simulink model "car_dynamics"  (R2023a)
settings: Solver=ode1be  StartTime=0.0  StopTime=100  FixedStep=0.01  RelTol=1e-4  AbsTol=1e-4
libraries: simulink_extras x3
settings Model: Creator=Sebas  LastModifiedBy=maxpr
settings SolverCC: AutoScaleAbsTol=off  SolverJacobianMethodControl=SparsePerturbation  AlgebraicLoopSolver=TrustRegion  EnableFixedStepZeroCrossing=on
settings OptimizationCC: ReuseModelBlockBuffer=off
settings DebuggingCC: UnconnectedInputMsg=warning  UnconnectedOutputMsg=warning  UnconnectedLineMsg=warning
settings ModelReferenceCC: EnableRefExpFcnMdlSchedulingChecks=on

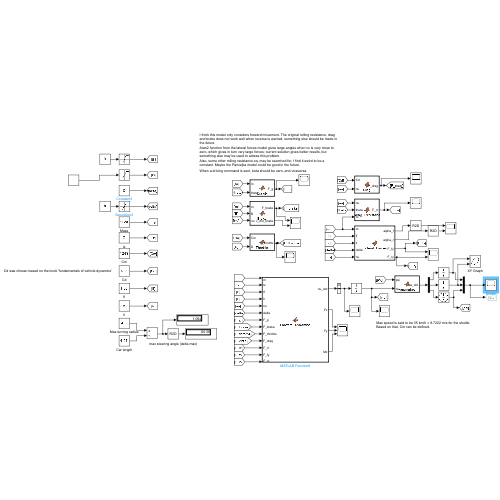
[thumbnail: Simulink's stored preview of the top-level diagram]
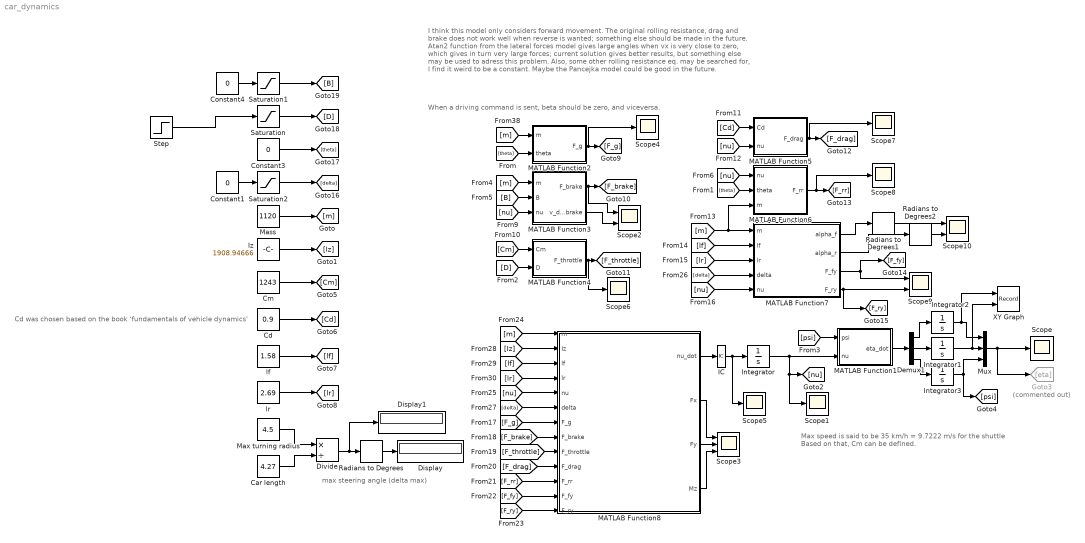
== system car_dynamics ==
  note: I think this model only considers forward movement. The original rolling resistance, drag and brake does not work well when reverse is wanted; something else should be made in the future.
      | Atan2 function from the lateral forces model gives large angles when vx is very close to zero, which gives in turn very large forces; current solution gives better results, but something else may be used to adress this problem.
      | Also, some other rolling resistance eq. may be searched for, I find it weird to be a constant. Maybe the Pancejka model could be good in the future.
  note: Max speed is said to be 35 km/h = 9.7222 m/s for the shuttle
      | Based on that, Cm can be defined.
  note: Cd was chosen based on the book 'fundamentals of vehicle dynamics'
  note: When a driving command is sent, beta should be zero, and viceversa.
  note: max steering angle (delta max)
  Car length : Constant  Value=4.27
  Cd : Constant  Value=0.9
  Cm : Constant  Value=1243
  Constant1 : Constant  Value=0
  Constant3 : Constant  Value=0
  Constant4 : Constant  Value=0
  Demux1 : Demux  Outputs=3
  Display : Display
  Display1 : Display
  Divide : Product  Inputs=*/
  Goto3 : Goto  Commented=on  GotoTag=eta
  IC : InitialCondition  Value=[0;0;0]
  Integrator : Integrator
  Integrator1 : Integrator
  Integrator2 : Integrator
  Integrator3 : Integrator  WrapState=on
  Iz : Constant  Value=1908.94666
  MATLAB Function1 : MATLAB Function  TreatAsAtomicUnit=on
  MATLAB Function2 : MATLAB Function  TreatAsAtomicUnit=on
  MATLAB Function3 : MATLAB Function  TreatAsAtomicUnit=on
  MATLAB Function4 : MATLAB Function  TreatAsAtomicUnit=on
  MATLAB Function5 : MATLAB Function  TreatAsAtomicUnit=on
  MATLAB Function6 : MATLAB Function  TreatAsAtomicUnit=on
  MATLAB Function7 : MATLAB Function  TreatAsAtomicUnit=on
  MATLAB Function8 : MATLAB Function  TreatAsAtomicUnit=on
  Mass : Constant  Value=1120
  Max turning radius : Constant  Value=4.5
  Mux : Mux  Inputs=3
  Radians to Degrees : simulink_extras/Transformations/Radians to Degrees
  Radians to Degrees1 : simulink_extras/Transformations/Radians to Degrees
  Radians to Degrees2 : simulink_extras/Transformations/Radians to Degrees
  Saturation : Saturate  UpperLimit=1  LowerLimit=0
  Saturation1 : Saturate  UpperLimit=1  LowerLimit=0
  Saturation2 : Saturate  UpperLimit=1.054  LowerLimit=-1.054
  Scope{,1,4..8} (7 alike) : Scope
  Scope10 : Scope  NumInputPorts=2
  Scope2 : Scope  NumInputPorts=2
  Scope3 : Scope  NumInputPorts=3
  Scope9 : Scope  NumInputPorts=2
  Step : Step  Time=50  Before=1  After=0  SampleTime=0
  XY Graph : Record  FileSettingsInternal="{\"entries\":[{\"content\":{\"excelSettings\":{\"content\":{},\"type\":\"Streamout.ExcelSettings\"}},\"type\":\"Streamout.FileSettingStorage\",\"uuid\":\"\"}],\"packageUris\":[\"http:\\/\\/schema.mathworks.com\\/mf0\\/streamout_blocks\\/R2020a\"],\"version\":\"1.0\"}"  Layout=[1 1]  SignalsInternal="{\"entries\":[{\"content\":{\"signals\":[{\"content\":{\"blockPath\":[],\"dimensions\":[1],\"domain\":\"\",\"lineColor\":\"#a2142f\",\"plots\":[1],\"port\":1,\"sid\":[\"\"],\"signalID\":582,\"signalName\":\"Integrator2\"},\"type\":\"RecordBlkView.Signal\",\"uuid\":\"\"},{\"content\":{\"blockPath\":[],\"dimensions\":[1],\"domain\":\"\",\"lineColor\":\"#139fff\",\"plots\":[1],\"port\":2,\"sid\":[\"\"],\"signalID\":586,\"signalName\":\"Integrator1\"},\"type\":\"RecordBlkView.Signal\",\"uuid\":\"\"}]},\"type\":\"RecordBlkView.InputSignals\",\"uuid\":\"\"}],\"packageUris\":[\"http:\\/\\/schema.mathworks.com\\/mf0\\/streamout_blocks\\/R2020a\"],\"version\":\"1.0\"}"  VisualizationBindings="{\"xyplotplugin\":{\"info\":[{\"series\":[{\"bindingParametersList\":[{\"parameter\":\"X-Axis\",\"signalID\":582,\"signalName\":\"Integrator2\"},{\"parameter\":\"Y-Axis\",\"signalID\":586,\"signalName\":\"Integrator1\"}],\"seriesID\":10362}],\"subplotID\":1}]}}"  CompatibilityTag=XY  st=-1
  lf : Constant  Value=1.58
  lr : Constant  Value=2.69
  wires:
  Max turning radius/1 -> Divide/1
  Car length/1 -> Divide/2
  Radians to Degrees/1 -> Display/1
  Divide/1 -> Display1/1, Radians to Degrees/1
  Iz/1 -> [Iz]
  Mass/1 -> [m]
  Cm/1 -> [Cm]
  Cd/1 -> [Cd]
  lr/1 -> [lr]
  lf/1 -> [lf]
  [theta] -> MATLAB Function2/2(theta)
  [m] -> MATLAB Function3/1(m)
  [nu] -> MATLAB Function3/3(nu)
  [Cm] -> MATLAB Function4/1(Cm)
  [Cd] -> MATLAB Function5/1(Cd)
  [nu] -> MATLAB Function5/2(nu)
  [lf] -> MATLAB Function7/2(lf)
  [lr] -> MATLAB Function7/3(lr)
  [delta] -> MATLAB Function7/4(delta)
  [nu] -> MATLAB Function7/5(nu)
  MATLAB Function2/1(F_g) -> Scope4/1, [F_g]
  MATLAB Function3/1(F_brake) -> Scope2/1, [F_brake]
  MATLAB Function4/1(F_throttle) -> Scope6/1, [F_throttle]
  MATLAB Function5/1(F_drag) -> Scope7/1, [F_drag]
  MATLAB Function6/1(F_rr) -> Scope8/1, [F_rr]
  MATLAB Function7/3(F_fy) -> [F_fy], Scope9/1
  MATLAB Function7/4(F_ry) -> Scope9/2, [F_ry]
  [F_g] -> MATLAB Function8/7(F_g)
  [F_brake] -> MATLAB Function8/8(F_brake)
  [F_throttle] -> MATLAB Function8/9(F_throttle)
  [F_drag] -> MATLAB Function8/10(F_drag)
  [F_rr] -> MATLAB Function8/11(F_rr)
  [F_fy] -> MATLAB Function8/12(F_fy)
  [F_ry] -> MATLAB Function8/13(F_ry)
  [m] -> MATLAB Function8/1(m)
  [nu] -> MATLAB Function8/5(nu)
  Constant1/1 -> Saturation2/1
  [delta] -> MATLAB Function8/6(delta)
  [Iz] -> MATLAB Function8/2(Iz)
  [lf] -> MATLAB Function8/3(lf)
  [lr] -> MATLAB Function8/4(lr)
  Integrator3/1 -> [psi], Mux/3
  Demux1/3 -> Integrator3/1
  Integrator1/1 -> XY Graph/2, Mux/2
  Mux/1 -> Goto3/1, Scope/1
  [psi] -> MATLAB Function1/1(psi)
  MATLAB Function1/1(eta_dot) -> Demux1/1
  Integrator/1 -> MATLAB Function1/2(nu), [nu], Scope1/1
  Integrator2/1 -> XY Graph/1, Mux/1
  Demux1/1 -> Integrator2/1
  IC/1 -> Scope5/1, Integrator/1
  Demux1/2 -> Integrator1/1
  MATLAB Function8/1(nu_dot) -> IC/1
  MATLAB Function8/2(Fx) -> Scope3/1
  MATLAB Function8/3(Fy) -> Scope3/2
  MATLAB Function8/4(Mz) -> Scope3/3
  [m] -> MATLAB Function2/1(m)
  [B] -> MATLAB Function3/2(B)
  MATLAB Function3/2(v_dot_brake) -> Scope2/2
  Saturation2/1 -> [delta]
  [m] -> MATLAB Function7/1(m), MATLAB Function6/3(m)
  Constant3/1 -> [theta]
  [theta] -> MATLAB Function6/2(theta)
  Constant4/1 -> Saturation1/1
  Saturation/1 -> [D]
  [D] -> MATLAB Function4/2(D)
  Saturation1/1 -> [B]
  [nu] -> MATLAB Function6/1(nu)
  MATLAB Function7/1(alpha_f) -> Radians to Degrees1/1
  MATLAB Function7/2(alpha_r) -> Radians to Degrees2/1
  Radians to Degrees1/1 -> Scope10/1
  Radians to Degrees2/1 -> Scope10/2
  Step/1 -> Saturation/1

== matlab function car_dynamics/MATLAB Function1 ==
  data: psi input; eta_dot output; nu input
function eta_dot = kinematics(psi, nu)
    R = [cos(psi) -sin(psi) 0;
         sin(psi) cos(psi) 0;
         0 0 1];
    
     eta_dot = R*nu;
end

== matlab function car_dynamics/MATLAB Function2 ==
  data: m input; theta input; F_g output
function F_g = Gravity(m,theta)
    % theta : vehicle pitch angle
    g = 9.81;
    
    F_g = m*g*sin(theta);
end

== matlab function car_dynamics/MATLAB Function3 ==
  data: m input; B input; F_brake output; nu input; v_dot_brake output
function [F_brake,v_dot_brake]= Brake(m,B,nu)
    % B : pedal brake command (or position) [0, 1]
    
    vx = nu(1);
    % If this condition is not set, the simulation breaks as velocities
    % tend to infinity
    if(vx > 0)
        % I don't think the original model consider reverse motion nor
        % standstill situations.
        % Moreover, this model could lend excesive forces. A simple test
        % was made with initial longitudinal velocity of 3 m/s and the
        % brake force was -800 N; it could be important to analyze this
        % furthermore.
        v_dot_brake = min(0,2.27-6.12*B+0.00535*vx);
    else
        v_dot_brake = 0;
    end

    F_brake = m*v_dot_brake;
end

== matlab function car_dynamics/MATLAB Function4 ==
  data: Cm input; F_throttle output; D input
function F_throttle = Throttle(Cm,D)
    % Cm : motor model constant
    % D : throttle command (or position) [0, 1]

    F_throttle = Cm*D;
end

== matlab function car_dynamics/MATLAB Function5 ==
  data: Cd input; F_drag output; nu input
function F_drag = Drag(Cd,nu)
    % D : throttle command (or position) [0, 1]
    % ro : air density
    % A : transversal area
    % Cd : drag coefficient

    vx = nu(1);
    ro = 1.225;
    A = 3.426;
    
    F_drag = 0.5*ro*A*Cd*vx^2;
end

== matlab function car_dynamics/MATLAB Function6 ==
  data: nu input; theta input; F_rr output; m input
function F_rr = Rolling_Resistance(nu,theta,m)
    % fr : rolling resistance coefficient

    fr = 0.038; % For passenger cars, from fundamentals of vehicle dynamics book

    % This resistance force does does not consider standstill
    % situations. If the vehicle is at rest, the car moves backwards
    F_rr = m*9.81*fr*cos(theta); % From fundamentals of vehicle dynamics book

end

== matlab function car_dynamics/MATLAB Function7 ==
  data: alpha_f output; alpha_r output; F_fy output; F_ry output; m input; lf input; lr input; delta input; nu input
function [alpha_f,alpha_r,F_fy, F_ry]= Lateral_Forces(m,lf,lr,delta,nu)
    % delta : steering angle
    % theta_vf : front tire velocity angle
    % theta_vr : rear tire velocity angle
    % C_alpha : tire cornering stiffness (assuming being equal for all tires)

    vx = nu(1);
    vy = nu(2);
    r = nu(3);

    % C alpha calculated from this webpage: https://www.mchenrysoftware.com/medit32/readme/msmac/default.htm?turl=examplestirecorneringstiffnesscalculation1.htm
    % Calculations made sense, as the Calpha of the Stanford Stanley car
    % are similar by being calculated with the same method
    C_alpha = m*9.81/2*0.165*57.2957; %N/rad

    alpha_f = atan2(vy + lf*r,vx) - delta;
    alpha_r = atan2(vy - lr*r,vx);

    if(vx > 0.01)
        % For some reason, atan2 was breaking the simulation in the integration
        % blocks using ode1 solver. By changing to ode14x or ode1b a better
        % response was acquired
        F_fy = -C_alpha*alpha_f;
        F_ry = -C_alpha*alpha_r;
    else
        F_fy = 0;
        F_ry = 0;
    end
end

== matlab function car_dynamics/MATLAB Function8 ==
  data: m input; Iz input; lf input; lr input; nu input; delta input; F_g input; nu_dot output; F_brake input; F_throttle input; F_drag input; F_rr input; F_fy input; F_ry input; Fx output; Fy output; Mz output
function [nu_dot,Fx,Fy,Mz]= Forward_Dynamics(m,Iz,lf,lr,nu,delta,F_g,F_brake,F_throttle,F_drag,F_rr,F_fy,F_ry)
    vx = nu(1);
    vy = nu(2);
    r = nu(3);
    
    % Next condition was set so the vehicle does not move backwards when
    % the throttle force is less than the resistance
    if(F_rr >= F_throttle && vx<0.01)
        F_rr = F_throttle;
    end
    Fx = F_brake + F_throttle - F_drag - F_rr - F_g - F_fy*sin(delta) + m*vy*r;
    Fy = F_ry + F_fy*cos(delta) - m*vx*r;
    Mz = F_fy*lf*cos(delta) - F_ry*lr;

    vx_dot = Fx/m;
    vy_dot = Fy/m;
    r_dot = Mz/Iz;
    
    nu_dot = [vx_dot;
             vy_dot;
             r_dot];
end
